simulink model "pacemaker"  (R2020a)
settings: Solver=FixedStepAuto  StartTime=0.0  StopTime=10.0  FixedStep=1e-3  RelTol=1e-3  EnableMultiTasking=on
undefined symbols (not defined in the file): A0, A1, D0, D1, D10, D11, D12, D13, D2, D3, D4, D5, D6, D7, D8, D9, PTA0, PTA1, PTA2, PTB2, PTB23, PTB3, PTB9, PTC16, PTC17, PTC2, PTC3, PTC4, PTD0, PTD1, PTD2, PTD3
libraries: frdmk64flib x20, etargetslib x7, dspstat3 x1
settings Model: ExtModeTrigDuration=5  Creator=safanaal-emara  LastModifiedBy=safanaal-emara
settings OptimizationCC: EnhancedBackFolding=on  PassReuseOutputArgsAs=Individual arguments  ZeroExternalMemoryAtStartup=off  ZeroInternalMemoryAtStartup=off  MaxStackSize=64  OptimizeBlockOrder=speed  DifferentSizesBufferReuse=on  OptimizationCustomize=off  EfficientTunableParamExpr=on
settings DebuggingCC: ParameterTunabilityLossMsg=error
settings HardwareCC: ProdBitPerPointer=32  ProdBitPerSizeT=32  ProdBitPerPtrDiffT=32  ProdLargestAtomicInteger=Long  ProdLargestAtomicFloat=Double  ProdWordSize=32  ProdHWDeviceType=ARM Compatible->ARM Cortex
settings SFSimCC: MATLABDynamicMemAlloc=off
settings RTWCC: SystemTargetFile=ert.tlc  HardwareBoard=NXP FRDM-K64F  TemplateMakefile=ert_default_tmf  Toolchain=GNU Tools for ARM Embedded Processors
settings CodeAppCC: ForceParamTrailComments=on  IgnoreCustomStorageClasses=off  OperatorAnnotations=on  SimulinkDataObjDesc=on  SFDataObjDesc=on  InsertBlockDesc=on

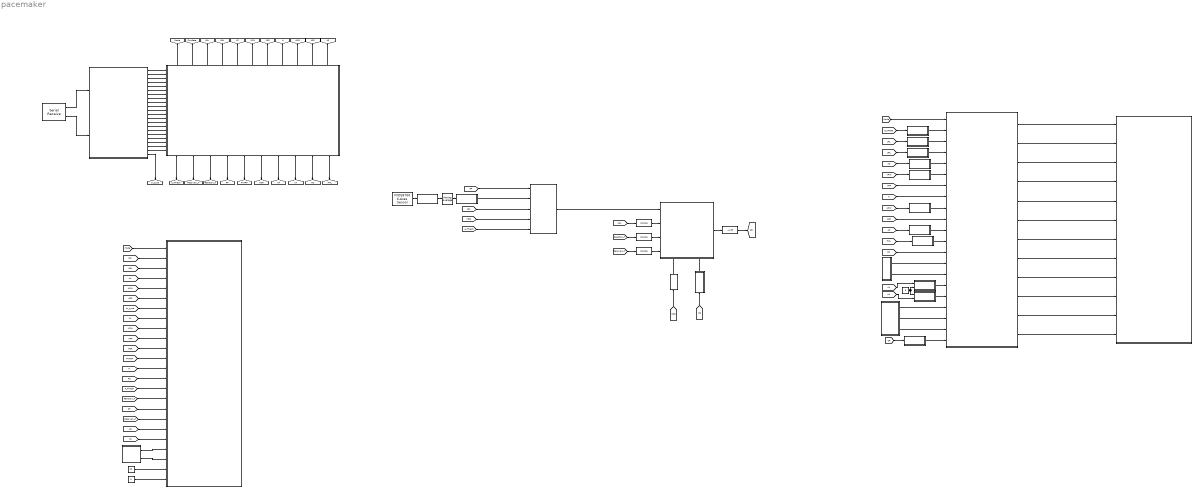
== system pacemaker ==
  note: MODES IMPLEMENTATION
  note: RATE ADAPTIVE PACING
  note: SERIAL COMMUNICATION
  AS : Subsystem
  Activity : Subsystem
  Adaptive : Stateflow chart  TreatAsAtomicUnit=on
      settings: PortSchema="{\"entries\":[{\"content\":{\"sides\":[{\"content\":{\"connectorIds\":[\"In1\",\"In2\",\"In3\",\"In4\"]},\"type\":\"ConnectorPlacement.EquallySpacedRectSide\",\"uuid\":\"fe050f22-06e5-4282-8c1f-2d2223b97801\"},{\"content\":{\"connectorIds\":[\"Out1\"],\"side\":\"RIGHT\"},\"type\":\"ConnectorPlacement.EquallySpacedRectSide\",\"uuid\":\"c3804d61-a816-4068-9373-d872d22aa45e\"},{\"content\":{\"connectorIds\":[],\"side\":\"TOP\"},\"type\":\"ConnectorPlacement.EquallySpacedRectSide\",\"uuid\":\"85dadf07-7824-4321-84a5-5a71239fb63c\"},{\"content\":{\"connectorIds\":[\"In5\",\"In6\"],\"side\":\"BOTTOM\"},\"type\":\"ConnectorPlacement.EquallySpacedRectSide\",\"uuid\":\"2d9ddbd1-241b-4ba1-84fc-026b5b263aab\"}]},\"type\":\"ConnectorPlacement.EquallySpacedConnector\",\"uuid\":\"413b58e1-2749-4ee4-a174-cb4eb9d57a26\"}],\"packageUris\":[\"http://schema.mathworks.com/mf0/Connector/19700101\"],\"version\":\"1.0\"}"
  COMM_IN : Stateflow chart  TreatAsAtomicUnit=on
      settings: PortSchema="{\"entries\":[{\"content\":{\"sides\":[{\"content\":{\"connectorIds\":[\"In1\",\"In2\"]},\"type\":\"ConnectorPlacement.EquallySpacedRectSide\",\"uuid\":\"6d8dc20d-05a6-41c0-8aa0-ece9a728cc0a\"},{\"content\":{\"connectorIds\":[\"Out1\",\"Out2\",\"Out3\",\"Out4\",\"Out5\",\"Out6\",\"Out7\",\"Out8\",\"Out9\",\"Out10\",\"Out11\",\"Out12\",\"Out13\",\"Out14\",\"Out15\",\"Out18\",\"Out16\",\"Out17\",\"Out19\",\"Out20\",\"Out22\",\"Out21\"],\"side\":\"RIGHT\"},\"type\":\"ConnectorPlacement.EquallySpacedRectSide\",\"uuid\":\"d43fa3b2-a7a8-4b43-9ceb-bf1dc59f8d01\"},{\"content\":{\"connectorIds\":[],\"side\":\"TOP\"},\"type\":\"ConnectorPlacement.EquallySpacedRectSide\",\"uuid\":\"bbed9bc0-4f6f-4f4c-9082-be73ecf4be5e\"}]},\"type\":\"ConnectorPlacement.EquallySpacedConnector\",\"uuid\":\"c2cc14cb-36b7-4132-be1a-3134ae9a24e5\"}],\"packageUris\":[\"http://schema.mathworks.com/mf0/Connector/19700101\"],\"version\":\"1.0\"}"
  Calculating DDC_A : Subsystem
  Calculating DDC_V : Subsystem
  Constant : Constant  Value=22  OutDataTypeStr=uint8
  Constant1 : Constant  Value=0
  Data Type Conversion{,1..3} (4 alike) : DataTypeConversion  OutDataTypeStr=double  RndMeth=Zero
  Data Type Conversion4 : DataTypeConversion  OutDataTypeStr=uint8  RndMeth=Ceiling
  Desired_Rate_Calc : Subsystem
  FXOS8700 6-Axes Sensor : frdmk64flib/FXOS8700 6-Axes Sensor  Activesensor=Accelerometer only  ODR=400Hz  HybridODR=400Hz  Accelfullrange=-4g to +4g  SampleTime=-1
  Function-Call Subsystem : Subsystem  TreatAsAtomicUnit=on
  HIGH/LOW : Subsystem
  INPUT : Subsystem
  INPUT1 : Subsystem
  MODES : Stateflow chart  TreatAsAtomicUnit=on
      settings: PortSchema="{\"entries\":[{\"content\":{\"sides\":[{\"content\":{\"connectorIds\":[\"In10\",\"In19\",\"In1\",\"In2\",\"In4\",\"In3\",\"In5\",\"In11\",\"In12\",\"In13\",\"In14\",\"In20\",\"In6\",\"In8\",\"In7\",\"In16\",\"In17\",\"In9\",\"In15\",\"In21\",\"In18\"]},\"type\":\"ConnectorPlacement.EquallySpacedRectSide\",\"uuid\":\"0889717d-8b09-4f94-9ffa-e6ec73606ec2\"},{\"content\":{\"connectorIds\":[\"Out11\",\"Out4\",\"Out1\",\"Out8\",\"Out10\",\"Out7\",\"Out9\",\"Out12\",\"Out5\",\"Out2\",\"Out6\",\"Out3\"],\"side\":\"RIGHT\"},\"type\":\"ConnectorPlacement.EquallySpacedRectSide\",\"uuid\":\"990f19e8-9bf0-4460-8f70-df74962d12f6\"},{\"content\":{\"connectorIds\":[],\"side\":\"TOP\"},\"type\":\"ConnectorPlacement.EquallySpacedRectSide\",\"uuid\":\"3670467e-f5bb-4ae2-af1a-ce21842cccd4\"}]},\"type\":\"ConnectorPlacement.EquallySpacedConnector\",\"uuid\":\"093de836-b894-432f-9081-ba9146477c25\"}],\"packageUris\":[\"http://schema.mathworks.com/mf0/Connector/19700101\"],\"version\":\"1.0\"}"
  Max_Voltage : Constant  Value=5
  Moving Average : dspstat3/Moving Average  Method=Sliding window  ForgettingFactorPort=off  SpecifyWindowLength=on  WindowLength=400  ForgettingFactor=0.9  SimulateUsing=Code generation
  OUTPUT : Subsystem
  Rate Smoothing : Subsystem
  Rate to ms : Subsystem
  Rate to ms 1 : Subsystem
  Rate to ms 2 : Subsystem
  Rate to ms 3 : Subsystem
  Rate to ms 5 : Subsystem
  SERIAL_FIX : Subsystem
  SERIAL_FIX2 : Subsystem
  Serial Receive : frdmk64flib/Serial Receive  SCIModule=0  Baudrate=uint32(9600)  Parity=None  StopBits=1  HardwareFlowControl=None  ByteOrder=LittleEndian  DataType=uint8  DataLength=43  BlockingMode=off  OutputStatus=on  SampleTime=-1
  Subsystem : Subsystem
  VS : Subsystem
  safety : Stateflow chart  TreatAsAtomicUnit=on
      settings: PortSchema="{\"entries\":[{\"content\":{\"sides\":[{\"content\":{\"connectorIds\":[\"In6\",\"In19\",\"In5\",\"In13\",\"In16\",\"In14\",\"In15\",\"In20\",\"In2\",\"In3\",\"In4\",\"In21\",\"In11\",\"In18\",\"In1\",\"In7\",\"In8\",\"In10\",\"In12\",\"In9\",\"In17\"]},\"type\":\"ConnectorPlacement.EquallySpacedRectSide\",\"uuid\":\"28f5cd87-14d2-468d-b30e-78b62bbd1f0e\"},{\"content\":{\"connectorIds\":[],\"side\":\"RIGHT\"},\"type\":\"ConnectorPlacement.EquallySpacedRectSide\",\"uuid\":\"4a0a5bf2-def2-410f-ba18-cf38f79986a1\"},{\"content\":{\"connectorIds\":[\"Out8\",\"Out19\",\"Out1\",\"Out3\",\"Out17\",\"Out15\",\"Out16\",\"Out20\",\"Out5\",\"Out6\",\"Out7\"],\"side\":\"TOP\"},\"type\":\"ConnectorPlacement.EquallySpacedRectSide\",\"uuid\":\"c3191ef5-bf84-4580-94cd-3213ace29dcc\"},{\"content\":{\"connectorIds\":[\"Out18\",\"Out10\",\"Out13\",\"Out11\",\"Out9\",\"Out2\",\"Out4\",\"Out14\",\"Out12\",\"Out21\"],\"side\":\"BOTTOM\"},\"type\":\"ConnectorPlacement.EquallySpacedRectSide\",\"uuid\":\"3ff6ffe3-1e7a-45a8-8169-9075f56b8f8a\"}]},\"type\":\"ConnectorPlacement.EquallySpacedConnector\",\"uuid\":\"70a0293d-52a4-448c-b9da-84157a3ae3b5\"}],\"packageUris\":[\"http://schema.mathworks.com/mf0/Connector/19700101\"],\"version\":\"1.0\"}"
  tag scope: AA=global, APW=global, ARP=global, AS=global, A_Thresh=global, CR=global, CurrRate=global, H=global, HRL=global, LRL=global, MSR=global, Mode=global, PVARP=global, RF=global, RS=global, Reaction_T=global, Recovery_T=global, URL=global, VA=global, VPW=global, VRP=global, VS=global, tx_type=global
  wires:
  Rate to ms 2/1(Out1) -> MODES/1(LRL)
  Rate to ms 5/1(Out1) -> MODES/20(HRL)
  Rate to ms 3/1(Out1) -> MODES/2(URL)
  Rate to ms/1(Out1) -> MODES/19(CurRate)
  MODES/11(ATR_CMP_REF_PWM) -> OUTPUT/1(In1)
  MODES/4(ATR_PACE_CTRL) -> OUTPUT/2(In2)
  MODES/1(ATR_GND_CTRL) -> OUTPUT/3(In3)
  MODES/8(Z_ATR_CTRL) -> OUTPUT/4(In4)
  MODES/10(VENT_PACE_CTRL) -> OUTPUT/5(In5)
  MODES/7(VENT_GND_CTRL) -> OUTPUT/6(In6)
  MODES/9(Z_VENT_CTRL) -> OUTPUT/7(In7)
  MODES/12(FRONTEND_CTRL) -> OUTPUT/8(In8)
  MODES/5(VENT_CMP_REF_PWM) -> OUTPUT/9(In9)
  MODES/2(PACE_CHARGE_CTRL) -> OUTPUT/10(In10)
  MODES/6(PACE_GND_CTRL) -> OUTPUT/11(In11)
  INPUT/1(Out1) -> MODES/9(VENT_CMP_DETECT)
  INPUT/2(Out2) -> MODES/15(ATR_CMP_DETECT)
  MODES/3(PACING_REF_PWM) -> OUTPUT/12(In12)
  Max_Voltage/1 -> Calculating DDC_A/1(In), Calculating DDC_V/2(In2)
  Calculating DDC_A/1(Out1) -> MODES/17(DDC_A)
  Calculating DDC_V/1(Out1) -> MODES/16(DDC_V)
  HIGH/LOW/2(Out2) -> MODES/7(HIGH)
  FXOS8700 6-Axes Sensor/1 -> Subsystem/1(In1)
  Subsystem/1(Out1) -> Moving Average/1
  Moving Average/1 -> Activity/1(In1)
  Desired_Rate_Calc/1(newbpms) -> Adaptive/1(DESIRED_RATE)
  Rate to ms 1/1(Out1) -> MODES/18(ACurRate)
  Rate Smoothing/1(Out1) -> Adaptive/6(RS)
  Activity/1(Activity) -> Desired_Rate_Calc/2(Activity)
  Serial Receive/2 -> COMM_IN/2(status)
  Serial Receive/1 -> COMM_IN/1(rx_data)
  [Mode] -> MODES/10(MODE)
  [CurrRate] -> Rate to ms/1(In1)
  [LRL] -> Rate to ms 2/1(In1)
  [URL] -> Rate to ms 3/1(In1)
  [VS] -> VS/1(In1)
  [VRP] -> MODES/5(VRP)
  [H] -> MODES/11(H)
  [HRL] -> Rate to ms 5/1(In1)
  [RS] -> MODES/6(RS)
  HIGH/LOW/1(Out1) -> MODES/8(LOW)
  [VA] -> Calculating DDC_V/1(In1)
  [AA] -> Calculating DDC_A/2(In1)
  [MSR] -> Desired_Rate_Calc/4(MSR)
  [LRL] -> Desired_Rate_Calc/3(LRL)
  [RF] -> Desired_Rate_Calc/1(RF)
  [A_Thresh] -> Desired_Rate_Calc/5(AThresh)
  [Mode] -> Function-Call Subsystem/1(Mode)
  [LRL] -> Function-Call Subsystem/2(LRL)
  [URL] -> Function-Call Subsystem/3(URL)
  [VA] -> Function-Call Subsystem/8(VA)
  [AA] -> Function-Call Subsystem/4(AA)
  [APW] -> Function-Call Subsystem/5(APW)
  [ARP] -> Function-Call Subsystem/6(ARP)
  [tx_type] -> Function-Call Subsystem/7(tx_type)
  [VPW] -> Function-Call Subsystem/9(VPW)
  [VRP] -> Function-Call Subsystem/10(VRP)
  [MSR] -> Function-Call Subsystem/11(MSR)
  [PVARP] -> Function-Call Subsystem/12(PVARP)
  [H] -> Function-Call Subsystem/13(H)
  [RS] -> Function-Call Subsystem/14(RS)
  [AS] -> Function-Call Subsystem/19(AS)
  [A_Thresh] -> Function-Call Subsystem/15(A_Thresh)
  [Reaction_T] -> Function-Call Subsystem/16(Reaction_T)
  [RF] -> Function-Call Subsystem/17(RF)
  [Recovery_T] -> Function-Call Subsystem/18(Recovery_T)
  INPUT1/1(Out1) -> Function-Call Subsystem/21(ATR_SIGNAL)
  INPUT1/2(Out2) -> Function-Call Subsystem/22(VENT_SIGNAL)
  [VS] -> Function-Call Subsystem/20(VS)
  Constant/1 -> Function-Call Subsystem/23(SYNC)
  [RS] -> Rate Smoothing/1(In1)
  [APW] -> SERIAL_FIX2/1(In1)
  SERIAL_FIX2/1(Out1) -> MODES/12(APW)
  [ARP] -> MODES/13(ARP)
  [VPW] -> SERIAL_FIX/1(In1)
  SERIAL_FIX/1(Out1) -> MODES/3(VPW)
  [CR] -> Rate to ms 1/1(In1)
  [LRL] -> Data Type Conversion3/1
  Data Type Conversion3/1 -> Adaptive/2(LRL)
  [Reaction_T] -> Data Type Conversion2/1
  Data Type Conversion2/1 -> Adaptive/3(RT)
  [Recovery_T] -> Data Type Conversion1/1
  Data Type Conversion1/1 -> Adaptive/4(RCT)
  Data Type Conversion/1 -> Adaptive/5(MSR)
  [MSR] -> Data Type Conversion/1
  Adaptive/1(CR) -> Data Type Conversion4/1
  Data Type Conversion4/1 -> [CR]
  [AS] -> AS/1(In1)
  AS/1(Out1) -> MODES/14(AS)
  VS/1(Out1) -> MODES/4(VS)
  INPUT/3(Out3) -> MODES/21(button)
  COMM_IN/1(Mode) -> safety/6(MODE)
  COMM_IN/15(AA) -> safety/1(AA)
  COMM_IN/18(MSR) -> safety/7(MSR)
  COMM_IN/19(Reaction_T) -> safety/12(RT)
  COMM_IN/20(Recovery_T) -> safety/9(RCT)
  COMM_IN/14(VA) -> safety/18(VA)
  COMM_IN/17(RF) -> safety/10(RF)
  COMM_IN/22(A_Thresh) -> safety/17(A_Thresh)
  COMM_IN/21(tx_type) -> [tx_type]
  COMM_IN/16(PVARP) -> safety/8(PVARP)
  COMM_IN/3(LRL) -> safety/5(LRL)
  COMM_IN/4(URL) -> safety/13(URL)
  COMM_IN/5(VS) -> safety/16(VS)
  COMM_IN/6(VPW) -> safety/14(VPW)
  COMM_IN/7(VRP) -> safety/15(VRP)
  COMM_IN/9(APW) -> safety/2(APW)
  COMM_IN/10(ARP) -> safety/3(ARP)
  COMM_IN/11(AS) -> safety/4(AS)
  COMM_IN/13(RS) -> safety/11(RS)
  COMM_IN/2(CurrRate) -> safety/19(CurRate)
  COMM_IN/8(H) -> safety/20(H)
  COMM_IN/12(HRL) -> safety/21(HRL)
  safety/21(hrl) -> [HRL]
  safety/12(rs) -> [RS]
  safety/14(va) -> [VA]
  safety/4(aa) -> [AA]
  safety/2(msr) -> [MSR]
  safety/9(pvarp) -> [PVARP]
  safety/11(rf) -> [RF]
  safety/13(rt) -> [Reaction_T]
  safety/10(rct) -> [Recovery_T]
  safety/18(a_Thresh) -> [A_Thresh]
  safety/8(mode) -> [Mode]
  safety/19(CurrRate) -> [CurrRate]
  safety/1(lrl) -> [LRL]
  safety/3(url) -> [URL]
  safety/17(vs) -> [VS]
  safety/15(vpw) -> [VPW]
  safety/16(vrp) -> [VRP]
  safety/20(h) -> [H]
  safety/5(apw) -> [APW]
  safety/6(arp) -> [ARP]
  safety/7(as) -> [AS]
  Constant1/1 -> Function-Call Subsystem/24(Input)

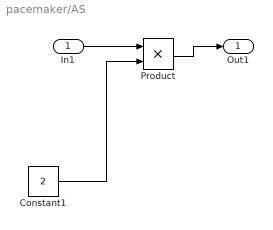
== system pacemaker/AS ==
  In1 : Inport
  Constant1 : Constant  Value=2
  Product : Product  OutDataTypeStr=uint8
  Out1 : Outport
  wires:
  In1/1 -> Product/1
  Constant1/1 -> Product/2
  Product/1 -> Out1/1

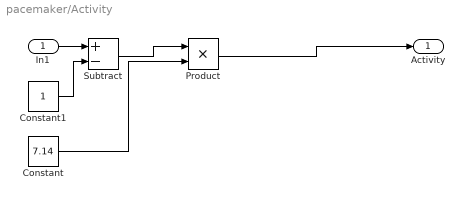
== system pacemaker/Activity ==
  In1 : Inport
  Constant : Constant  Value=7.14
  Constant1 : Constant
  Product : Product
  Subtract : Sum  Inputs=+-
  Activity : Outport
  wires:
  Constant/1 -> Product/2
  Product/1 -> Activity/1
  Constant1/1 -> Subtract/2
  In1/1 -> Subtract/1
  Subtract/1 -> Product/1

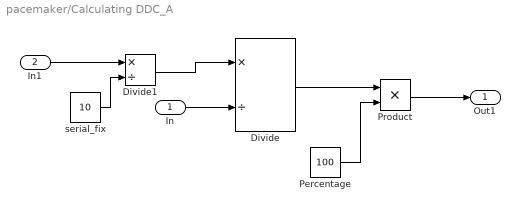
== system pacemaker/Calculating DDC_A ==
  In : Inport
  In1 : Inport  Port=2
  Divide : Product  Inputs=*/
  Divide1 : Product  Inputs=*/
  Percentage : Constant  Value=100
  Product : Product
  serial_fix : Constant  Value=10
  Out1 : Outport
  wires:
  In/1 -> Divide/2
  In1/1 -> Divide1/1
  Product/1 -> Out1/1
  Divide/1 -> Product/1
  Percentage/1 -> Product/2
  Divide1/1 -> Divide/1
  serial_fix/1 -> Divide1/2

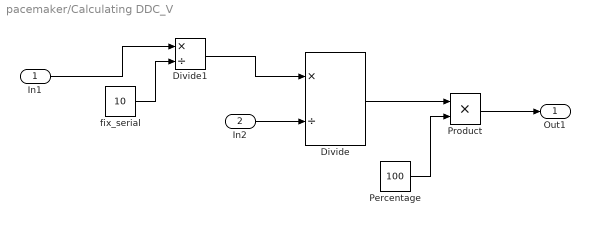
== system pacemaker/Calculating DDC_V ==
  In1 : Inport
  In2 : Inport  Port=2
  Divide : Product  Inputs=*/
  Divide1 : Product  Inputs=*/
  Percentage : Constant  Value=100
  Product : Product
  fix_serial : Constant  Value=10
  Out1 : Outport
  wires:
  In2/1 -> Divide/2
  In1/1 -> Divide1/1
  Product/1 -> Out1/1
  Divide/1 -> Product/1
  Percentage/1 -> Product/2
  Divide1/1 -> Divide/1
  fix_serial/1 -> Divide1/2

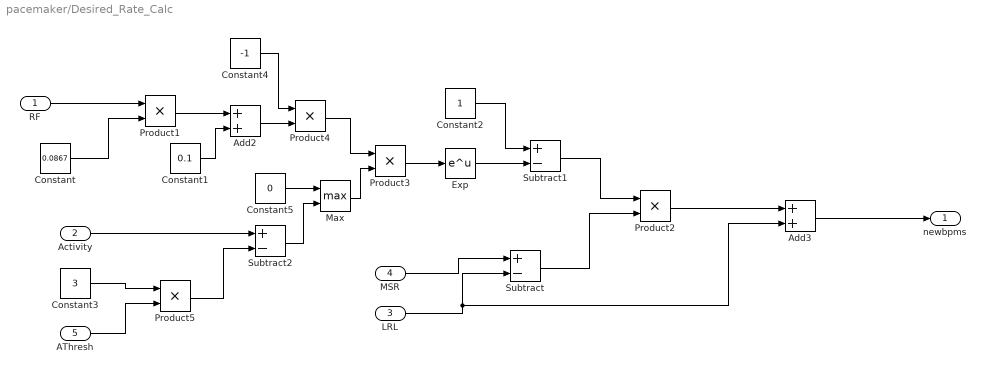
== system pacemaker/Desired_Rate_Calc ==
  RF : Inport
  Activity : Inport  Port=2
  LRL : Inport  Port=3
  MSR : Inport  Port=4
  AThresh : Inport  Port=5
  Add2 : Sum
  Add3 : Sum  OutDataTypeStr=double  RndMeth=Zero
  Constant : Constant  Value=0.0867
  Constant1 : Constant  Value=0.1
  Constant2 : Constant
  Constant3 : Constant  Value=3
  Constant4 : Constant  Value=-1
  Constant5 : Constant  Value=0
  Exp : Math  SaturateOnIntegerOverflow=on
  Max : MinMax  Function=max  Inputs=2
  Product{1..5} (5 alike) : Product
  Subtract : Sum  Inputs=+-
  Subtract1 : Sum  Inputs=+-
  Subtract2 : Sum  Inputs=+-
  newbpms : Outport
  wires:
  Constant3/1 -> Product5/1
  Product5/1 -> Subtract2/2
  Subtract1/1 -> Product2/1
  AThresh/1 -> Product5/2
  Subtract/1 -> Product2/2
  Subtract2/1 -> Max/2
  Max/1 -> Product3/2
  MSR/1 -> Subtract/1
  Exp/1 -> Subtract1/2
  Product2/1 -> Add3/1
  Constant4/1 -> Product4/1
  Add2/1 -> Product4/2
  Product1/1 -> Add2/1
  Constant/1 -> Product1/2
  Activity/1 -> Subtract2/1
  RF/1 -> Product1/1
  Product3/1 -> Exp/1
  Constant5/1 -> Max/1
  Constant1/1 -> Add2/2
  Product4/1 -> Product3/1
  Constant2/1 -> Subtract1/1
  LRL/1 -> Add3/2, Subtract/2
  Add3/1 -> newbpms/1

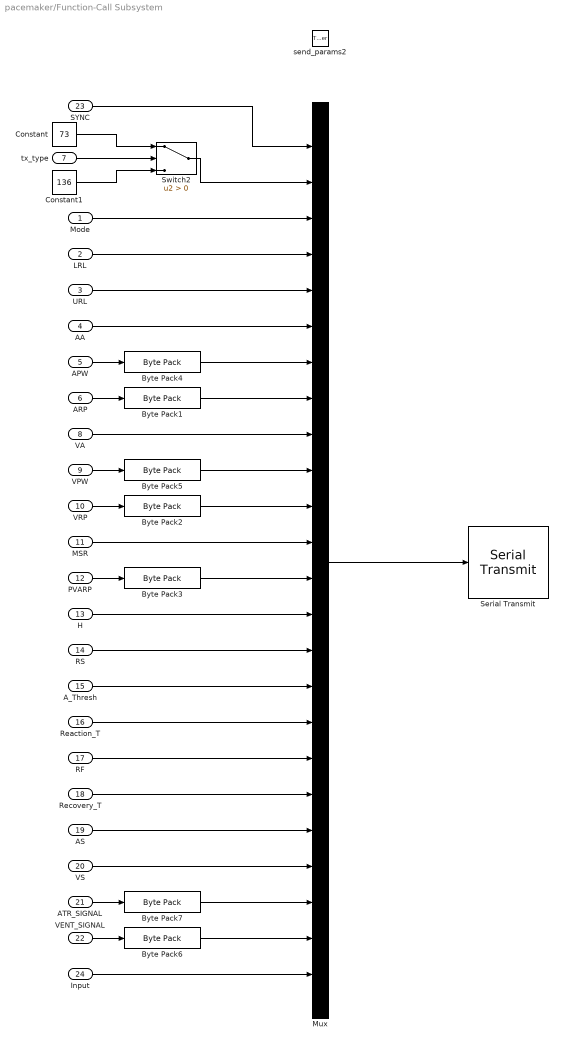
== system pacemaker/Function-Call Subsystem ==
  Mode : Inport
  LRL : Inport  Port=2
  URL : Inport  Port=3
  AA : Inport  Port=4
  APW : Inport  Port=5
  ARP : Inport  Port=6
  tx_type : Inport  Port=7
  VA : Inport  Port=8
  VPW : Inport  Port=9
  VRP : Inport  Port=10
  MSR : Inport  Port=11
  PVARP : Inport  Port=12
  H : Inport  Port=13
  RS : Inport  Port=14
  A_Thresh : Inport  Port=15
  Reaction_T : Inport  Port=16
  RF : Inport  Port=17
  Recovery_T : Inport  Port=18
  AS : Inport  Port=19
  VS : Inport  Port=20
  ATR_SIGNAL : Inport  Port=21
  VENT_SIGNAL : Inport  Port=22
  SYNC : Inport  Port=23
  Input : Inport  Port=24
  send_params2 : TriggerPort  TriggerType=function-call  IsSimulinkFunction=on  FunctionName=send_params2  VariantControl=Variant
  Byte Pack{1..5} (5 alike) : etargetslib/Byte Pack  datatypes={'uint16'}  byteAlign=1
  Byte Pack6 : etargetslib/Byte Pack  datatypes={'double'}  byteAlign=1
  Byte Pack7 : etargetslib/Byte Pack  datatypes={'double'}  byteAlign=1
  Constant : Constant  Value=73  OutDataTypeStr=uint8
  Constant1 : Constant  Value=136  OutDataTypeStr=uint8
  Mux : Mux  Inputs=24
  Serial Transmit : frdmk64flib/Serial Transmit  SCIModule=0  Baudrate=uint32(9600)  Parity=None  StopBits=1  HardwareFlowControl=None  ByteOrder=LittleEndian  BlockingMode=on  OutputStatus=off
  Switch2 : Switch  Criteria=u2 > Threshold
  wires:
  ARP/1 -> Byte Pack1/1
  VRP/1 -> Byte Pack2/1
  tx_type/1 -> Switch2/2
  Mux/1 -> Serial Transmit/1
  PVARP/1 -> Byte Pack3/1
  VS/1 -> Mux/21
  AS/1 -> Mux/20
  Recovery_T/1 -> Mux/19
  RF/1 -> Mux/18
  Reaction_T/1 -> Mux/17
  A_Thresh/1 -> Mux/16
  RS/1 -> Mux/15
  H/1 -> Mux/14
  Byte Pack3/1 -> Mux/13
  MSR/1 -> Mux/12
  Byte Pack2/1 -> Mux/11
  Byte Pack1/1 -> Mux/8
  URL/1 -> Mux/5
  LRL/1 -> Mux/4
  SYNC/1 -> Mux/1
  Mode/1 -> Mux/3
  Switch2/1 -> Mux/2
  Constant/1 -> Switch2/1
  Constant1/1 -> Switch2/3
  Input/1 -> Mux/24
  VENT_SIGNAL/1 -> Byte Pack6/1
  Byte Pack6/1 -> Mux/23
  Byte Pack7/1 -> Mux/22
  ATR_SIGNAL/1 -> Byte Pack7/1
  AA/1 -> Mux/6
  VA/1 -> Mux/9
  APW/1 -> Byte Pack4/1
  Byte Pack4/1 -> Mux/7
  VPW/1 -> Byte Pack5/1
  Byte Pack5/1 -> Mux/10

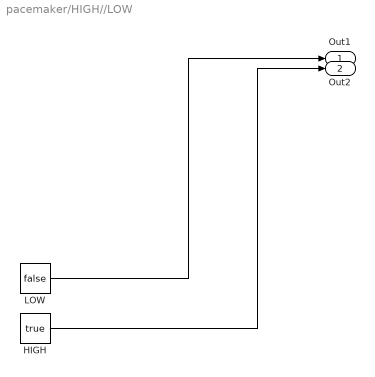
== system pacemaker/HIGH//LOW ==
  HIGH : Constant  Value=true
  LOW : Constant  Value=false
  Out1 : Outport
  Out2 : Outport  Port=2
  wires:
  HIGH/1 -> Out2/1
  LOW/1 -> Out1/1

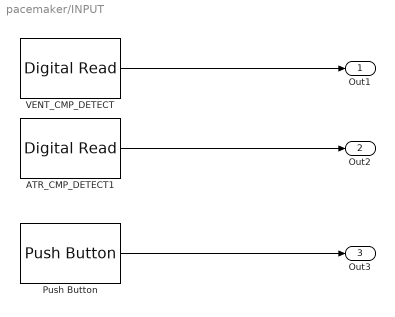
== system pacemaker/INPUT ==
  ATR_CMP_DETECT1 : frdmk64flib/Digital Read  Whichpin=PTC16 (D0)  SampleTime=0.001
  Push Button : frdmk64flib/Push Button  Whichswitch=SW2  SampleTime1=-1
  VENT_CMP_DETECT : frdmk64flib/Digital Read  Whichpin=PTC17 (D1)  SampleTime=0.001
  Out1 : Outport
  Out2 : Outport  Port=2
  Out3 : Outport  Port=3
  wires:
  VENT_CMP_DETECT/1 -> Out1/1
  ATR_CMP_DETECT1/1 -> Out2/1
  Push Button/1 -> Out3/1

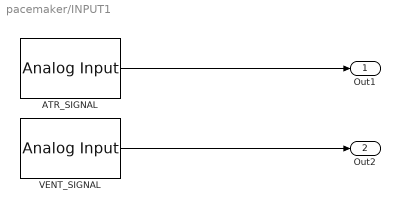
== system pacemaker/INPUT1 ==
  ATR_SIGNAL : frdmk64flib/Analog Input  Whichpin=PTB2 (A0)  SampleTime=-1
  VENT_SIGNAL : frdmk64flib/Analog Input  Whichpin=PTB3 (A1)  SampleTime=-1
  Out1 : Outport  OutDataTypeStr=double
  Out2 : Outport  Port=2  OutDataTypeStr=double
  wires:
  ATR_SIGNAL/1 -> Out1/1
  VENT_SIGNAL/1 -> Out2/1

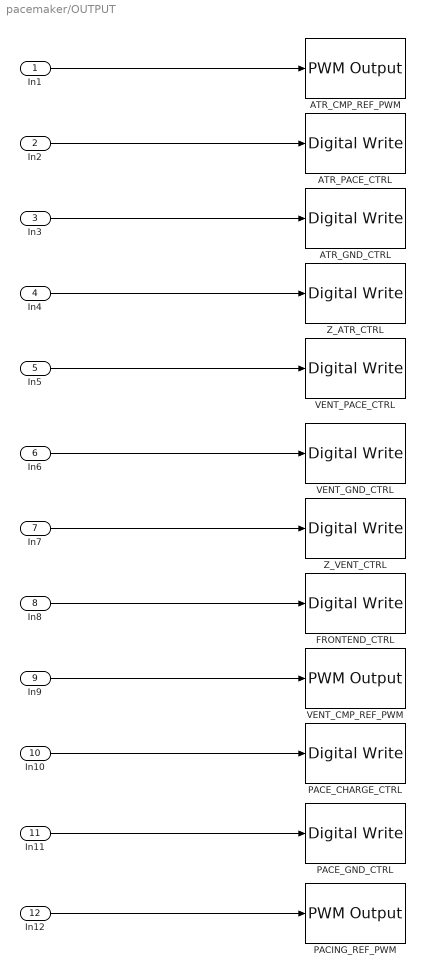
== system pacemaker/OUTPUT ==
  In1 : Inport
  In2 : Inport  Port=2
  In3 : Inport  Port=3
  In4 : Inport  Port=4
  In5 : Inport  Port=5
  In6 : Inport  Port=6
  In7 : Inport  Port=7
  In8 : Inport  Port=8
  In9 : Inport  Port=9
  In10 : Inport  Port=10
  In11 : Inport  Port=11
  In12 : Inport  Port=12
  ATR_CMP_REF_PWM : frdmk64flib/PWM Output  Whichpin=PTC2 (D6)  InitialFrequency=2000  InitialDutyCycle=20
  ATR_GND_CTRL : frdmk64flib/Digital Write  Whichpin=PTD2 (D11)
  ATR_PACE_CTRL : frdmk64flib/Digital Write  Whichpin=PTA0 (D8)
  FRONTEND_CTRL : frdmk64flib/Digital Write  Whichpin=PTD1 (D13)
  PACE_CHARGE_CTRL : frdmk64flib/Digital Write  Whichpin=PTB9 (D2)
  PACE_GND_CTRL : frdmk64flib/Digital Write  Whichpin=PTD0 (D10)
  PACING_REF_PWM : frdmk64flib/PWM Output  Whichpin=PTA2 (D5)  InitialFrequency=2000  InitialDutyCycle=100
  VENT_CMP_REF_PWM : frdmk64flib/PWM Output  Whichpin=PTA1 (D3)  InitialFrequency=2000  InitialDutyCycle=20
  VENT_GND_CTRL : frdmk64flib/Digital Write  Whichpin=PTD3 (D12)
  VENT_PACE_CTRL : frdmk64flib/Digital Write  Whichpin=PTC4 (D9)
  Z_ATR_CTRL : frdmk64flib/Digital Write  Whichpin=PTB23 (D4)
  Z_VENT_CTRL : frdmk64flib/Digital Write  Whichpin=PTC3 (D7)
  wires:
  In1/1 -> ATR_CMP_REF_PWM/1
  In2/1 -> ATR_PACE_CTRL/1
  In3/1 -> ATR_GND_CTRL/1
  In4/1 -> Z_ATR_CTRL/1
  In5/1 -> VENT_PACE_CTRL/1
  In6/1 -> VENT_GND_CTRL/1
  In7/1 -> Z_VENT_CTRL/1
  In8/1 -> FRONTEND_CTRL/1
  In9/1 -> VENT_CMP_REF_PWM/1
  In10/1 -> PACE_CHARGE_CTRL/1
  In11/1 -> PACE_GND_CTRL/1
  In12/1 -> PACING_REF_PWM/1

== system pacemaker/Rate Smoothing ==
  In1 : Inport
  Constant : Constant  Value=100000
  Divide : Product  Inputs=*/  OutDataTypeStr=double  RndMeth=Zero
  Out1 : Outport
  wires:
  In1/1 -> Divide/1
  Constant/1 -> Divide/2
  Divide/1 -> Out1/1

== system pacemaker/Rate to ms ==
  In1 : Inport
  Constant : Constant  Value=30000
  Divide : Product  Inputs=*/  OutDataTypeStr=uint16  RndMeth=Ceiling
  Out1 : Outport
  wires:
  In1/1 -> Divide/2
  Constant/1 -> Divide/1
  Divide/1 -> Out1/1

== system pacemaker/Rate to ms 1 ==
  In1 : Inport
  Constant : Constant  Value=30000
  Divide : Product  Inputs=*/  OutDataTypeStr=uint16  RndMeth=Ceiling
  Out1 : Outport
  wires:
  In1/1 -> Divide/2
  Constant/1 -> Divide/1
  Divide/1 -> Out1/1

== system pacemaker/Rate to ms 2 ==
  In1 : Inport
  Constant : Constant  Value=30000
  Divide : Product  Inputs=*/  OutDataTypeStr=uint16  RndMeth=Ceiling
  Out1 : Outport
  wires:
  In1/1 -> Divide/2
  Constant/1 -> Divide/1
  Divide/1 -> Out1/1

== system pacemaker/Rate to ms 3 ==
  In1 : Inport
  Constant : Constant  Value=30000
  Divide : Product  Inputs=*/  OutDataTypeStr=uint16  RndMeth=Ceiling
  Out1 : Outport
  wires:
  In1/1 -> Divide/2
  Constant/1 -> Divide/1
  Divide/1 -> Out1/1

== system pacemaker/Rate to ms 5 ==
  In1 : Inport
  Constant : Constant  Value=30000
  Divide : Product  Inputs=*/  OutDataTypeStr=uint16  RndMeth=Ceiling
  Out1 : Outport
  wires:
  In1/1 -> Divide/2
  Constant/1 -> Divide/1
  Divide/1 -> Out1/1

== system pacemaker/SERIAL_FIX ==
  In1 : Inport
  Divide : Product  Inputs=*/  OutDataTypeStr=double  RndMeth=Zero
  serial_fix : Constant  Value=10
  Out1 : Outport
  wires:
  In1/1 -> Divide/1
  Divide/1 -> Out1/1
  serial_fix/1 -> Divide/2

== system pacemaker/SERIAL_FIX2 ==
  In1 : Inport
  Divide : Product  Inputs=*/  OutDataTypeStr=double  RndMeth=Zero
  serial_fix : Constant  Value=10
  Out1 : Outport
  wires:
  In1/1 -> Divide/1
  Divide/1 -> Out1/1
  serial_fix/1 -> Divide/2

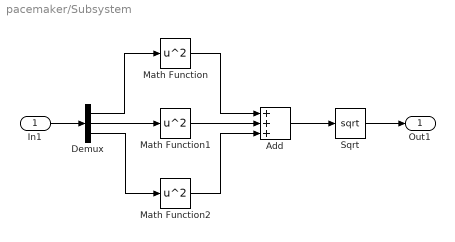
== system pacemaker/Subsystem ==
  In1 : Inport
  Add : Sum  Inputs=+++
  Demux : Demux  Outputs=3
  Math Function : Math  Operator=square  SaturateOnIntegerOverflow=on
  Math Function1 : Math  Operator=square  SaturateOnIntegerOverflow=on
  Math Function2 : Math  Operator=square  SaturateOnIntegerOverflow=on
  Sqrt : Sqrt  SaturateOnIntegerOverflow=on
  Out1 : Outport
  wires:
  In1/1 -> Demux/1
  Demux/1 -> Math Function/1
  Demux/2 -> Math Function1/1
  Demux/3 -> Math Function2/1
  Math Function/1 -> Add/1
  Math Function1/1 -> Add/2
  Math Function2/1 -> Add/3
  Add/1 -> Sqrt/1
  Sqrt/1 -> Out1/1

== system pacemaker/VS ==
  In1 : Inport
  Constant1 : Constant  Value=2
  Product : Product  OutDataTypeStr=uint8
  Out1 : Outport
  wires:
  In1/1 -> Product/1
  Constant1/1 -> Product/2
  Product/1 -> Out1/1

== stateflow chart pacemaker/Adaptive ==
  state STEPUP
    entry:
    if(stepup/CR>RS && RS~=0)
    CR=(1+2*RS)*CR
    else
    CR=CR+(2*stepup);
    end
  state DEFAULT
    during:
    CR=LRL;
    stepup=((MSR-LRL)/RT)/1000;
    stepdown=((MSR-LRL)/(RCT  ))/1000;
  state MAINTAIN
    entry:
    CR=DESIRED_RATE
  state STANDBY
    entry:
  state STEPDOWN
    entry:
    if(stepdown/CR>RS && RS~=0)
    CR=(1-2*RS)*CR
    else
    CR=CR-(2*stepdown);
    end
  STEPUP -> STEPUP [order 1] : [after(2,msec)]
  (default) -> DEFAULT
  STEPUP -> MAINTAIN [order 2] : [(CR-(2*stepup))<DESIRED_RATE&&(CR+(2*stepup))>DESIRED_RATE]
  DEFAULT -> STEPUP : [DESIRED_RATE>LRL]
  MAINTAIN -> STEPUP [order 1] : [CR<DESIRED_RATE]
  STEPUP -> STANDBY [order 3] : [(CR-stepup)>DESIRED_RATE]
  (junction 79) -> STEPUP [order 1] : [CR<DESIRED_RATE]
  STANDBY -> (junction 79) : [after(1000, msec)]
  (junction 79) -> STEPDOWN [order 2] : [CR>DESIRED_RATE]
  STEPDOWN -> STANDBY [order 3] : [(CR+stepdown)<DESIRED_RATE]
  MAINTAIN -> STEPDOWN [order 2] : [CR>DESIRED_RATE]
  STEPDOWN -> MAINTAIN [order 2] : [(CR-(2*stepdown))<DESIRED_RATE&&(CR+(2*stepdown))>DESIRED_RATE]
  STEPDOWN -> STEPDOWN [order 1] : [after(2, msec)]
  data: DESIRED_RATE input; LRL input; RT input; CR output; RCT input; MSR input; RS input; stepdown local; stepup local

== stateflow chart pacemaker/COMM_IN ==
  settings: executeAtInitialization=1
  state UPDATE_PARAMS
    % Update params from DCM
    entry:
    Mode = typecast(rx_data(3), 'uint8');
    LRL = typecast(rx_data(4), 'uint8');
    CurrRate = typecast(rx_data(4), 'uint8');
    URL = typecast(rx_data(5), 'uint8');
    AA = typecast(rx_data(6),'uint8');
    APW = typecast(rx_data(7:8), 'uint16');
    ARP = typecast(rx_data(9:10), 'uint16');
    VA = typecast(rx_data(11),'uint8');
    VPW = typecast(rx_data(12:13), 'uint16');
    VRP = typecast(rx_data(14:15), 'uint16');
    MSR = typecast(rx_data(16),'uint8');
    PVARP = typecast(rx_data(17:18), 'uint16'); % NOT sure about this one
    H = typecast(rx_data(19),'uint8');
    RS = typecast(rx_data(20),'uint8');
    A_Thresh = typecast(rx_data(21),'uint8');
    Reaction_T = typecast(rx_data(22),'uint8');
    RF = typecast(rx_data(23),'uint8');
    Recovery_T = typecast(rx_data(24),'uint8');
    AS = typecast(rx_data(25),'uint8');
    VS = typecast(rx_data(26),'uint8');
    HRL = typecast(rx_data(4), 'uint8'); %% NOT SENT BY DCM
  state INITIAL
    % Set default values for parameters
    entry:
    Mode = 1;
    CurrRate = 60;
    LRL = 60;
    URL = 120;
    VS = 40;
    VPW = 4;
    VRP = 320;
    H = 0;
    APW = 4;
    ARP = 250;
    AS = 40;
    HRL = 60;
    RS = 0;
    VA = 35;
    AA = 35;
    MSR = 120;
    PVARP = 250;
    A_Thresh = 1;
    Reaction_T = 10;
    RF = 16;
    Recovery_T = 20;
  state STANDBY
    % Waiting for new data from DCM
  state SEND_PARAMS
    entry:
    tx_type = 1;
    send_params2();
  state SEND_EGRAM
    entry:
    tx_type = 0;
    send_params2();
  UPDATE_PARAMS -> STANDBY
  (default) -> INITIAL
  (junction 25) -> STANDBY [order 2]
  (junction 46) -> UPDATE_PARAMS [order 1] : [rx_data(2) == hex2dec('55')]
  INITIAL -> STANDBY
  STANDBY -> (junction 25) : [status == 0]
  (junction 25) -> (junction 46) [order 1] : [rx_data(1) == hex2dec('16')]
  (junction 46) -> SEND_EGRAM [order 3] : [rx_data(2) == hex2dec('47')]
  (junction 46) -> SEND_PARAMS [order 2] : [rx_data(2) == hex2dec('49')]
  SEND_EGRAM -> STANDBY
  SEND_PARAMS -> STANDBY
  data: Mode output uint8; CurrRate output uint8; LRL output uint8; URL output uint8; VS output uint8; VPW output uint16; VRP output uint16; H output uint8; APW output uint16; ARP output uint16; AS output uint8; HRL output uint8; RS output uint8; VA output uint8; rx_data input uint8; status input uint8; AA output uint8; PVARP output uint16; RF output uint8; MSR output uint8; Reaction_T output uint8; Recovery_T output uint8; tx_type output uint8; A_Thresh output uint8

== stateflow chart pacemaker/MODES ==
  state VVI
    state INIT
      entry:
      FRONTEND_CTRL=HIGH;
      VENT_CMP_REF_PWM=VS;
      countDown=CurRate;
      H_local=LOW;
    state VRP
      entry:
      VRPcount = VRP;
      during:
      VRPcount = VRPcount - 1;
    state SENSE
      during:
      countDown = countDown - 1;
    state HYSTERESIS
      entry:
      hyst_wait=HRL-CurRate;
      countDown=CurRate;
      during:
      if (H==LOW)
      hyst_wait=0;
      else
      hyst_wait = hyst_wait - 1;
      end
    state CHARGING_C22_DISCHARGING_C21
      entry:
      ATR_PACE_CTRL=LOW;
      VENT_PACE_CTRL=LOW;
      PACING_REF_PWM=DDC_V;
      PACE_CHARGE_CTRL=HIGH;
      PACE_GND_CTRL=HIGH;
      Z_ATR_CTRL=LOW;
      Z_VENT_CTRL=LOW;
      ATR_GND_CTRL=LOW;
      VENT_GND_CTRL=HIGH;
    state DISCHARGING_C22_AV
      entry:
      PACE_CHARGE_CTRL=LOW;
      PACE_GND_CTRL=HIGH;
      ATR_PACE_CTRL=LOW;
      ATR_GND_CTRL=LOW;
      Z_ATR_CTRL=LOW;
      Z_VENT_CTRL=LOW;
      VENT_GND_CTRL=LOW;
      VENT_PACE_CTRL=HIGH;
      PACING_REF_PWM=DDC_V;
    VVI.HYSTERESIS -> VVI.VRP [order 2] : [VENT_CMP_DETECT==HIGH]{H_local=HIGH}
    (default) -> VVI.INIT
    VVI.INIT -> VVI.SENSE
    VVI.SENSE -> VVI.HYSTERESIS [order 3] : [H_local== HIGH && VENT_CMP_DETECT==LOW && countDown<=0]
    VVI.VRP -> VVI.SENSE : [VRPcount<=0]{countDown = countDown-VRP}
    VVI.SENSE -> VVI.VRP [order 1] : [VENT_CMP_DETECT==HIGH]{countDown=CurRate, H_local=HIGH}
    VVI.DISCHARGING_C22_AV -> VVI.VRP
    VVI.SENSE -> VVI.CHARGING_C22_DISCHARGING_C21 [order 2] : [VENT_CMP_DETECT==LOW && countDown<=0 && H_local==LOW]{countDown=CurRate, H_local}
    VVI.HYSTERESIS -> VVI.CHARGING_C22_DISCHARGING_C21 [order 1] : [VENT_CMP_DETECT==LOW && hyst_wait<=0]{H_local=LOW}
    VVI.CHARGING_C22_DISCHARGING_C21 -> VVI.DISCHARGING_C22_AV : [after(VPW,msec)]{countDown=countDown-VPW}
  state AOO
    state CHARGING_C22_DISCHARGING_BLOCKING_CAP
      entry:
      ATR_PACE_CTRL=LOW;
      VENT_PACE_CTRL=LOW;
      PACING_REF_PWM=DDC_A;
      PACE_CHARGE_CTRL=HIGH;
      PACE_GND_CTRL=HIGH;
      Z_ATR_CTRL=LOW;
      Z_VENT_CTRL=LOW;
      ATR_GND_CTRL=HIGH;
      VENT_GND_CTRL=LOW;
    state DISCHARGING_C22
      entry:
      PACE_CHARGE_CTRL=LOW;
      PACE_GND_CTRL=HIGH;
      ATR_PACE_CTRL=HIGH;
      ATR_GND_CTRL=LOW;
      Z_ATR_CTRL=LOW;
      Z_VENT_CTRL=LOW;
      VENT_GND_CTRL=LOW;
      VENT_PACE_CTRL=LOW;
      PACING_REF_PWM=DDC_A;
    AOO.CHARGING_C22_DISCHARGING_BLOCKING_CAP -> AOO.DISCHARGING_C22 : [after((CurRate-APW),msec)]
    (default) -> AOO.CHARGING_C22_DISCHARGING_BLOCKING_CAP
    AOO.DISCHARGING_C22 -> AOO.CHARGING_C22_DISCHARGING_BLOCKING_CAP : [after(APW,msec)]
  state DEFAULT
    entry:
  state VOO
    state CHARGING_C22_DISCHARGING_BLOCKING_CAP
      entry:
      ATR_PACE_CTRL=LOW;
      VENT_PACE_CTRL=LOW;
      PACING_REF_PWM=DDC_V;
      PACE_CHARGE_CTRL=HIGH;
      PACE_GND_CTRL=HIGH;
      Z_ATR_CTRL=LOW;
      Z_VENT_CTRL=LOW;
      ATR_GND_CTRL=LOW;
      VENT_GND_CTRL=HIGH;
    state DISCHARGING_C22
      entry:
      PACE_CHARGE_CTRL=LOW;
      PACE_GND_CTRL=HIGH;
      ATR_PACE_CTRL=LOW;
      ATR_GND_CTRL=LOW;
      Z_ATR_CTRL=LOW;
      Z_VENT_CTRL=LOW;
      VENT_GND_CTRL=LOW;
      VENT_PACE_CTRL=HIGH;
      PACING_REF_PWM=DDC_V;
    VOO.CHARGING_C22_DISCHARGING_BLOCKING_CAP -> VOO.DISCHARGING_C22 : [after((CurRate-VPW),msec)]
    (default) -> VOO.CHARGING_C22_DISCHARGING_BLOCKING_CAP
    VOO.DISCHARGING_C22 -> VOO.CHARGING_C22_DISCHARGING_BLOCKING_CAP : [after(VPW,msec)]
  state AAI
    state INIT
      entry:
      FRONTEND_CTRL=HIGH;
      ATR_CMP_REF_PWM=AS;
      countDown=CurRate;
      H_local=LOW;
    state ARP
      entry:
      ARPcount = ARP;
      during:
      ARPcount = ARPcount - 1;
    state SENSE
      during:
      countDown = countDown - 1;
    state HYSTERESIS
      entry:
      hyst_wait=HRL-CurRate;
      countDown=CurRate;
      during:
      if (H==LOW)
      hyst_wait=0;
      else
      hyst_wait = hyst_wait - 1;
      end
    state CHARGING_C22_DISCHARGING_BLOCKING_CAP
      entry:
      ATR_PACE_CTRL=LOW;
      VENT_PACE_CTRL=LOW;
      PACING_REF_PWM=DDC_A;
      PACE_CHARGE_CTRL=HIGH;
      PACE_GND_CTRL=HIGH;
      Z_ATR_CTRL=LOW;
      Z_VENT_CTRL=LOW;
      ATR_GND_CTRL=HIGH;
      VENT_GND_CTRL=LOW;
    state DISCHARGING_C22
      entry:
      PACE_CHARGE_CTRL=LOW;
      PACE_GND_CTRL=HIGH;
      ATR_PACE_CTRL=HIGH;
      ATR_GND_CTRL=LOW;
      Z_ATR_CTRL=LOW;
      Z_VENT_CTRL=LOW;
      VENT_GND_CTRL=LOW;
      VENT_PACE_CTRL=LOW;
      PACING_REF_PWM=DDC_A;
    AAI.HYSTERESIS -> AAI.ARP [order 2] : [ATR_CMP_DETECT==HIGH]{H_local=HIGH}
    (default) -> AAI.INIT
    AAI.INIT -> AAI.SENSE
    AAI.SENSE -> AAI.HYSTERESIS [order 3] : [H_local== HIGH && ATR_CMP_DETECT==LOW && countDown<=0]
    AAI.ARP -> AAI.SENSE : [ARPcount<=0]{countDown = countDown-ARP}
    AAI.SENSE -> AAI.ARP [order 1] : [ATR_CMP_DETECT==HIGH]{countDown=CurRate, H_local=HIGH}
    AAI.DISCHARGING_C22 -> AAI.ARP
    AAI.SENSE -> AAI.CHARGING_C22_DISCHARGING_BLOCKING_CAP [order 2] : [ATR_CMP_DETECT==LOW && countDown<=0 && H_local==LOW]{countDown=CurRate, H_local}
    AAI.HYSTERESIS -> AAI.CHARGING_C22_DISCHARGING_BLOCKING_CAP [order 1] : [ATR_CMP_DETECT==LOW && hyst_wait<=0]{H_local=LOW}
    AAI.CHARGING_C22_DISCHARGING_BLOCKING_CAP -> AAI.DISCHARGING_C22 : [after(APW,msec)]{countDown=countDown-APW}
  state DDDR
    state INIT
      entry:
      %%Initialize variables
      FRONTEND_CTRL = HIGH;
      VAescape=ACurRate*8/10;
      AVD=ACurRate*2/10;
      ATR_CMP_REF_PWM = AS;
      VENT_CMP_REF_PWM = VS;
    state ATR_CHARGE
      entry:
      ATR_PACE_CTRL=LOW;
      VENT_PACE_CTRL=LOW;
      PACING_REF_PWM=DDC_A;
      PACE_CHARGE_CTRL=HIGH;
      PACE_GND_CTRL=HIGH;
      Z_ATR_CTRL=LOW;
      Z_VENT_CTRL=LOW;
      ATR_GND_CTRL=HIGH;
      VENT_GND_CTRL=LOW;
    state ATR_DISCHARGE
      entry:
      PACE_CHARGE_CTRL=LOW;
      PACE_GND_CTRL=HIGH;
      ATR_PACE_CTRL=HIGH;
      ATR_GND_CTRL=LOW;
      Z_ATR_CTRL=LOW;
      Z_VENT_CTRL=LOW;
      VENT_GND_CTRL=LOW;
      VENT_PACE_CTRL=LOW;
      PACING_REF_PWM=DDC_A;
    state ATR_SENSE
      entry:
    state VENT_CHARGE
      entry:
      ATR_PACE_CTRL=LOW;
      VENT_PACE_CTRL=LOW;
      PACING_REF_PWM=DDC_V;
      PACE_CHARGE_CTRL=HIGH;
      PACE_GND_CTRL=HIGH;
      Z_ATR_CTRL=LOW;
      Z_VENT_CTRL=LOW;
      ATR_GND_CTRL=LOW;
      VENT_GND_CTRL=HIGH;
    state VENT_DISCHARGE
      entry:
      PACE_CHARGE_CTRL=LOW;
      PACE_GND_CTRL=HIGH;
      ATR_PACE_CTRL=LOW;
      ATR_GND_CTRL=LOW;
      Z_ATR_CTRL=LOW;
      Z_VENT_CTRL=LOW;
      VENT_GND_CTRL=LOW;
      VENT_PACE_CTRL=HIGH;
      PACING_REF_PWM=DDC_V;
    state VENT_SENSE
      entry:
    VENT_DISCHARGE -> DDDR.INIT
    (default) -> DDDR.INIT
    VENT_SENSE -> DDDR.INIT [order 2] : [VENT_CMP_DETECT==HIGH || button == HIGH]
    DDDR.INIT -> ATR_SENSE
    ATR_SENSE -> ATR_CHARGE [order 1] : [after(VAescape, msec) && ATR_CMP_DETECT==LOW]
    ATR_CHARGE -> ATR_DISCHARGE : [after((APW),msec)]
    ATR_DISCHARGE -> VENT_SENSE
    ATR_SENSE -> VENT_SENSE [order 2] : [ATR_CMP_DETECT==HIGH]
    VENT_SENSE -> VENT_CHARGE [order 1] : [after(AVD, msec) && VENT_CMP_DETECT==LOW]
    VENT_CHARGE -> VENT_DISCHARGE : [after((VPW),msec)]
  state VOOR
    state CHARGING_C22_DISCHARGING_BLOCKING_CAP
      entry:
      ATR_PACE_CTRL=LOW;
      VENT_PACE_CTRL=LOW;
      PACING_REF_PWM=DDC_V;
      PACE_CHARGE_CTRL=HIGH;
      PACE_GND_CTRL=HIGH;
      Z_ATR_CTRL=LOW;
      Z_VENT_CTRL=LOW;
      ATR_GND_CTRL=LOW;
      VENT_GND_CTRL=HIGH;
    state DISCHARGING_C22
      entry:
      PACE_CHARGE_CTRL=LOW;
      PACE_GND_CTRL=HIGH;
      ATR_PACE_CTRL=LOW;
      ATR_GND_CTRL=LOW;
      Z_ATR_CTRL=LOW;
      Z_VENT_CTRL=LOW;
      VENT_GND_CTRL=LOW;
      VENT_PACE_CTRL=HIGH;
      PACING_REF_PWM=DDC_V;
    VOOR.CHARGING_C22_DISCHARGING_BLOCKING_CAP -> VOOR.DISCHARGING_C22 : [after((ACurRate-VPW),msec)]
    (default) -> VOOR.CHARGING_C22_DISCHARGING_BLOCKING_CAP
    VOOR.DISCHARGING_C22 -> VOOR.CHARGING_C22_DISCHARGING_BLOCKING_CAP : [after(VPW,msec)]
  state AAIR
    state INIT
      entry:
      FRONTEND_CTRL=HIGH;
      ATR_CMP_REF_PWM=AS;
      countDown= ACurRate;
      H_local=LOW;
    state ARP
      entry:
      ARPcount = ARP;
      during:
      ARPcount = ARPcount - 1;
    state SENSE
      during:
      countDown = countDown - 1;
    state HYSTERESIS
      entry:
      hyst_wait=HRL-ACurRate;
      countDown=ACurRate;
      during:
      if (H==LOW)
      hyst_wait=0;
      else
      hyst_wait = hyst_wait - 1;
      end
    state CHARGING_C22_DISCHARGING_BLOCKING_CAP
      entry:
      ATR_PACE_CTRL=LOW;
      VENT_PACE_CTRL=LOW;
      PACING_REF_PWM=DDC_A;
      PACE_CHARGE_CTRL=HIGH;
      PACE_GND_CTRL=HIGH;
      Z_ATR_CTRL=LOW;
      Z_VENT_CTRL=LOW;
      ATR_GND_CTRL=HIGH;
      VENT_GND_CTRL=LOW;
    state DISCHARGING_C22
      entry:
      PACE_CHARGE_CTRL=LOW;
      PACE_GND_CTRL=HIGH;
      ATR_PACE_CTRL=HIGH;
      ATR_GND_CTRL=LOW;
      Z_ATR_CTRL=LOW;
      Z_VENT_CTRL=LOW;
      VENT_GND_CTRL=LOW;
      VENT_PACE_CTRL=LOW;
      PACING_REF_PWM=DDC_A;
    AAIR.HYSTERESIS -> AAIR.ARP [order 2] : [ATR_CMP_DETECT==HIGH]{H_local=HIGH}
    (default) -> AAIR.INIT
    AAIR.INIT -> AAIR.SENSE
    AAIR.SENSE -> AAIR.HYSTERESIS [order 3] : [H_local== HIGH && ATR_CMP_DETECT==LOW && countDown<=0]
    AAIR.ARP -> AAIR.SENSE : [ARPcount<=0]{countDown = countDown-ARP}
    AAIR.SENSE -> AAIR.ARP [order 1] : [ATR_CMP_DETECT==HIGH]{countDown=ACurRate, H_local=HIGH}
    AAIR.DISCHARGING_C22 -> AAIR.ARP
    AAIR.SENSE -> AAIR.CHARGING_C22_DISCHARGING_BLOCKING_CAP [order 2] : [ATR_CMP_DETECT==LOW && countDown<=0 && H_local==LOW]{countDown=ACurRate, H_local}
    AAIR.HYSTERESIS -> AAIR.CHARGING_C22_DISCHARGING_BLOCKING_CAP [order 1] : [ATR_CMP_DETECT==LOW && hyst_wait<=0]{H_local=LOW}
    AAIR.CHARGING_C22_DISCHARGING_BLOCKING_CAP -> AAIR.DISCHARGING_C22 : [after(APW,msec)]{countDown=countDown-APW}
  state VVIR
    state INIT
      entry:
      FRONTEND_CTRL=HIGH;
      VENT_CMP_REF_PWM=VS;
      countDown=ACurRate;
      H_local=LOW;
    state VRP
      entry:
      VRPcount = VRP;
      during:
      VRPcount = VRPcount - 1;
    state SENSE
      during:
      countDown = countDown - 1;
    state HYSTERESIS
      entry:
      hyst_wait=HRL-ACurRate;
      countDown=ACurRate;
      during:
      if (H==LOW)
      hyst_wait=0;
      else
      hyst_wait = hyst_wait - 1;
      end
    state CHARGING_C22_DISCHARGING_C21
      entry:
      ATR_PACE_CTRL=LOW;
      VENT_PACE_CTRL=LOW;
      PACING_REF_PWM=DDC_V;
      PACE_CHARGE_CTRL=HIGH;
      PACE_GND_CTRL=HIGH;
      Z_ATR_CTRL=LOW;
      Z_VENT_CTRL=LOW;
      ATR_GND_CTRL=LOW;
      VENT_GND_CTRL=HIGH;
    state DISCHARGING_C22_AV
      entry:
      PACE_CHARGE_CTRL=LOW;
      PACE_GND_CTRL=HIGH;
      ATR_PACE_CTRL=LOW;
      ATR_GND_CTRL=LOW;
      Z_ATR_CTRL=LOW;
      Z_VENT_CTRL=LOW;
      VENT_GND_CTRL=LOW;
      VENT_PACE_CTRL=HIGH;
      PACING_REF_PWM=DDC_V;
    VVIR.HYSTERESIS -> VVIR.VRP [order 2] : [VENT_CMP_DETECT==HIGH]{H_local=HIGH}
    (default) -> VVIR.INIT
    VVIR.INIT -> VVIR.SENSE
    VVIR.SENSE -> VVIR.HYSTERESIS [order 3] : [H_local== HIGH && VENT_CMP_DETECT==LOW && countDown<=0]
    VVIR.VRP -> VVIR.SENSE : [VRPcount<=0]{countDown = countDown-VRP}
    VVIR.SENSE -> VVIR.VRP [order 1] : [VENT_CMP_DETECT==HIGH]{countDown=ACurRate, H_local=HIGH}
    VVIR.DISCHARGING_C22_AV -> VVIR.VRP
    VVIR.SENSE -> VVIR.CHARGING_C22_DISCHARGING_C21 [order 2] : [VENT_CMP_DETECT==LOW && countDown<=0 && H_local==LOW]{countDown=ACurRate, H_local}
    VVIR.HYSTERESIS -> VVIR.CHARGING_C22_DISCHARGING_C21 [order 1] : [VENT_CMP_DETECT==LOW && hyst_wait<=0]{H_local=LOW}
    VVIR.CHARGING_C22_DISCHARGING_C21 -> VVIR.DISCHARGING_C22_AV : [after(VPW,msec)]{countDown=countDown-VPW}
  state AOOR
    state CHARGING_C22_DISCHARGING_BLOCKING_CAP
      entry:
      ATR_PACE_CTRL=LOW;
      VENT_PACE_CTRL=LOW;
      PACING_REF_PWM=DDC_A;
      PACE_CHARGE_CTRL=HIGH;
      PACE_GND_CTRL=HIGH;
      Z_ATR_CTRL=LOW;
      Z_VENT_CTRL=LOW;
      ATR_GND_CTRL=HIGH;
      VENT_GND_CTRL=LOW;
    state DISCHARGING_C22
      entry:
      PACE_CHARGE_CTRL=LOW;
      PACE_GND_CTRL=HIGH;
      ATR_PACE_CTRL=HIGH;
      ATR_GND_CTRL=LOW;
      Z_ATR_CTRL=LOW;
      Z_VENT_CTRL=LOW;
      VENT_GND_CTRL=LOW;
      VENT_PACE_CTRL=LOW;
      PACING_REF_PWM=DDC_A;
    AOOR.CHARGING_C22_DISCHARGING_BLOCKING_CAP -> AOOR.DISCHARGING_C22 : [after((ACurRate-APW),msec)]
    (default) -> AOOR.CHARGING_C22_DISCHARGING_BLOCKING_CAP
    AOOR.DISCHARGING_C22 -> AOOR.CHARGING_C22_DISCHARGING_BLOCKING_CAP : [after(APW,msec)]
  DEFAULT -> VVI [order 1] : [MODE==3]
  AOO -> DEFAULT : [MODE~=2]
  DEFAULT -> AOO [order 3] : [MODE==2]
  VVI -> DEFAULT : [MODE~=3]
  (default) -> DEFAULT
  VOO -> DEFAULT : [MODE>1]
  DEFAULT -> VOO [order 2] : [MODE<=1]
  DDDR -> DEFAULT : [MODE~=9]
  DEFAULT -> DDDR [order 9] : [MODE==9]
  DEFAULT -> AAI [order 4] : [MODE==4]
  DEFAULT -> AAIR [order 7] : [MODE==8]
  AAI -> DEFAULT : [MODE~=4]
  VOOR -> DEFAULT : [MODE ~= 5]
  DEFAULT -> VOOR [order 5] : [MODE == 5]
  DEFAULT -> AOOR [order 8] : [MODE == 6]
  AOOR -> DEFAULT : [MODE~=6]
  DEFAULT -> VVIR [order 6] : [MODE==7]
  VVIR -> DEFAULT : [MODE~=7]
  AAIR -> DEFAULT : [MODE~=8]
  data: LRL input; URL input; VPW input; VS input; VRP input; RS input; HIGH input; LOW input; VENT_CMP_DETECT input; ATR_GND_CTRL output; PACE_CHARGE_CTRL output; PACING_REF_PWM output; ATR_PACE_CTRL output; VENT_CMP_REF_PWM output; PACE_GND_CTRL output; VENT_GND_CTRL output; Z_ATR_CTRL output; Z_VENT_CTRL output; VENT_PACE_CTRL output; countDown local; VRPcount local; H_local local; MODE input; H input; ARPcount local; APW input; ARP input; AS input; ATR_CMP_DETECT input; ATR_CMP_REF_PWM output; FRONTEND_CTRL output; hyst_wait local; VA constant double; DDC_V input; DDC_A input; RT local; ACurRate input; CurRate input; HRL input; AVD local; VAescape local; button input

== stateflow chart pacemaker/safety ==
  state DEFAULT
    entry:
    if 0 <= MODE <= 9
    mode=MODE;
    else
    mode=0;
    end
    if 50 <= LRL <= 90
    lrl = LRL
    CurrRate=LRL
    hrl=LRL
    else
    lrl = 60
    CurrRate=60
    hrl=60
    end
    if 50 <= URL <= 175
    url = URL
    else
    url =120
    end
    if lrl>url
    url = max(lrl, url);
    lrl = min(lrl, url);
    CurrRate=lrl;
    hrl=lrl;
    end
    if 50 <= MSR <= 175
    msr=MSR
    else
    msr=120
    end
    if lrl>msr
    msr = max(lrl, msr);
    lrl = min(lrl, msr);
    CurrRate=lrl
    hrl=lrl
    end
    if 0<= H <=1
    h=H
    else
    h=0
    end
    if 1<=AA<=50 %given as multiplied by 10 by DCM
    aa=AA
    else
    aa=35
    end
    if 1<=VA<=50 %given as multiplied by 10 by DCM
    va=VA
    else
    VA =35
    end
    if 10 <= APW <= 300 %given as multiplied by 10 by DCM
    apw=APW
    else
    apw=1
    end
    if 10<= VPW <= 300 %given as multiplied by 10 by DCM
    vpw=VPW
    else
    vpw=10
    end
    if 0 <= AS <= 50 %given as multiplied by 10 by DCM
    as=AS
    else
    as=35
    end
    if 0 <= VS <= 50 %given as multiplied by 10 by DCM
    vs=VS
    else
    vs=35
    end
    if 150 <= VRP <= 500
    vrp = VRP
    else
    vrp=320
    end
    if 150 <= ARP <= 500
    arp = ARP
    else
    arp=250
    end
    if 150 <= PVARP <= 500
    pvarp = PVARP
    else
    pvarp =250
    end
    if 0 <= RS <= 25
    rs=RS
    else
    rs=0
    end
    if 1 <= A_Thresh <= 7
    a_Thresh= A_Thresh
    else
    a_Thresh=1
    end
    if 10<RT<50
    rt=RT
    else
    rt=10
    end
    if 1<= RF <= 16
    rf=RF
    else
    rf=16
    end
    if 2 <= RCT <= 16
    rct=RCT
    else
    rct=2
    end
  (default) -> DEFAULT
  data: lrl output; msr output; url output; AA input; APW input; ARP input; AS input; LRL input; MODE input; MSR input; PVARP input; RCT input; RF input; RS input; RT input; URL input; VPW input; VRP input; VS input; A_Thresh input; aa output; apw output; arp output; as output; mode output; pvarp output; rct output; rf output; rs output; rt output; va output; vpw output; vrp output; vs output; VA input; a_Thresh output; CurRate input; CurrRate output; H input; h output; HRL input; hrl output
